simulink model "sampleModel2120_pp_532_1"  (R2021a)
settings: Solver=VariableStepAuto  StartTime=0.0  StopTime=10.0  RelTol=1e-3
undefined symbols (not defined in the file or in its folder): DiscIntNeverNeededParam, magnitude, Newton, Raphson
libraries: simulink x67, pid_lib x12
(part 2 of 3)

== system sampleModel2120_pp_532_1/emi_27 ==
  emi_34 : Inport
  Action Port : ActionPort  ActionPortLabel=if(0 > u1)
  emi_31 : Trigonometry
  emi_32 : Math  SaturateOnIntegerOverflow=on
  emi_33 : Gain
  emi_35 : Outport
  wires:
  emi_34/1 -> emi_31/1
  emi_31/1 -> emi_32/1
  emi_32/1 -> emi_33/1

== system sampleModel2120_pp_532_1/emi_45 ==
  emi_52 : Inport
  Action Port : ActionPort  ActionPortLabel=if(0 > u1)
  emi_49 : Trigonometry
  emi_50 : Abs
  emi_51 : Trigonometry
  emi_53 : Outport
  wires:
  emi_52/1 -> emi_49/1
  emi_49/1 -> emi_50/1
  emi_50/1 -> emi_51/1

== system sampleModel2120_pp_532_1/emi_6 ==
  emi_13 : Inport
  Action Port : ActionPort  ActionPortLabel=if(-1.783329e+09 > u1)
  emi_10 : Abs
  emi_11 : Gain
  emi_12 : Abs
  emi_14 : Outport
  wires:
  emi_13/1 -> emi_10/1
  emi_10/1 -> emi_11/1
  emi_11/1 -> emi_12/1

== system sampleModel2120_pp_532_1/emi_66 ==
  emi_73 : Inport
  Action Port : ActionPort  ActionPortLabel=if(0 > u1)
  emi_70 : Gain
  emi_71 : Math  SaturateOnIntegerOverflow=on
  emi_72 : Trigonometry
  emi_74 : Outport
  wires:
  emi_73/1 -> emi_70/1
  emi_70/1 -> emi_71/1
  emi_71/1 -> emi_72/1

== system sampleModel2120_pp_532_1/emi_90 ==
  emi_97 : Inport
  Action Port : ActionPort  ActionPortLabel=if(0 > u1)
  emi_94 : Abs
  emi_95 : Gain
  emi_96 : Trigonometry
  emi_98 : Outport
  wires:
  emi_97/1 -> emi_94/1
  emi_94/1 -> emi_95/1
  emi_95/1 -> emi_96/1

== system sampleModel2120_pp_532_1/cfblk45/cfblk10 ==
  cfblk1 : Inport
  cfblk10 : Sum  Inputs=+  OutDataTypeStr=double
  cfblk11 : Bias  Bias=[143732452.396222]
  cfblk3 : DiscreteFir  SampleTime=1
  cfblk4 : simulink/Discrete/Transfer Fcn Real Zero  ZeroZ=0.75  ICPrevInput=0.0  DoSatur=off
      settings: SourceProductBaseCode=SL
  cfblk5 : simulink/Discrete/Transfer Fcn First Order  PoleZ=0.95  ICPrevOutput=0.0  DoSatur=off
  cfblk6 : Delay  DelayLengthSource=Input port  SampleTime=1
      settings: InputPortMap=u0,p1
  cfblk7 : Bias  Bias=[415695908.441253]
  cfblk8 : simulink/Math Operations/Slider Gain  gain=1  low=0  high=2
  cfblk9 : Rounding
  cyemi_{24..33} (10 alike) : DataTypeConversion  OutDataTypeStr=double
  cfblk2 : Outport
  wires:
  cfblk9/1 -> cfblk2/1
  cfblk11/1 -> cyemi_26/1, cyemi_30/1
  cyemi_24/1 -> cfblk10/1
  cfblk5/1 -> cyemi_24/1
  cyemi_25/1 -> cfblk11/1
  cfblk8/1 -> cyemi_25/1
  cyemi_26/1 -> cfblk3/1
  cyemi_27/1 -> cfblk4/1
  cfblk3/1 -> cyemi_27/1
  cyemi_28/1 -> cfblk5/1
  cfblk4/1 -> cyemi_28/1
  cyemi_29/1 -> cfblk6/1
  cfblk10/1 -> cyemi_29/1
  cyemi_30/1 -> cfblk6/2
  cyemi_31/1 -> cfblk7/1
  cfblk1/1 -> cyemi_31/1
  cyemi_32/1 -> cfblk8/1
  cfblk7/1 -> cyemi_32/1
  cyemi_33/1 -> cfblk9/1
  cfblk6/1 -> cyemi_33/1

== system sampleModel2120_pp_532_1/cfblk45/cfblk11 ==
  cfblk1 : Inport
  cfblk6 : Inport  Port=2
  cfblk7 : Inport  Port=3
  cfblk8 : Inport  Port=4
  cfblk9 : Inport  Port=5
  cfblk3 : Sum  Inputs=-+  OutDataTypeStr=double
  cfblk4 : Constant  Value=[-156405987.882864]  OutDataTypeStr=double  SampleTime=1
  cfblk5 : Constant  Value=[-751982074.552397]  OutDataTypeStr=double  SampleTime=1
  cyemi_39 : DataTypeConversion  OutDataTypeStr=double
  cyemi_40 : DataTypeConversion  OutDataTypeStr=double
  cfblk2 : Outport
  cfblk10 : Outport  Port=2
  wires:
  cfblk4/1 -> cfblk10/1
  cfblk5/1 -> cfblk2/1
  cyemi_39/1 -> cfblk3/1
  cfblk8/1 -> cyemi_39/1
  cyemi_40/1 -> cfblk3/2
  cfblk7/1 -> cyemi_40/1

== system sampleModel2120_pp_532_1/cfblk45/cfblk12 ==
  cfblk1 : Inport
  cfblk11 : Inport  Port=2
  cfblk10 : Constant  Value=[257671330.793710]  OutDataTypeStr=double  SampleTime=1
  cfblk12 : Delay  SampleTime=1
  cfblk3 : simulink/Discrete/Transfer Fcn First Order  PoleZ=0.95  ICPrevOutput=0.0  DoSatur=off
  cfblk4 : Delay  ShowEnablePort=on  SampleTime=1
      settings: InputPortMap=u0,e6
  cfblk5 : DiscreteFilter  SampleTime=1
  cfblk6 : Product  OutDataTypeStr=double
  cfblk7 : Sum  Inputs=--  OutDataTypeStr=double
  cfblk8 : Sum  OutDataTypeStr=double
  cfblk9 : Constant  Value=[-533370526.019482]  OutDataTypeStr=double  SampleTime=1
  cyemi_{43..53} (11 alike) : DataTypeConversion  OutDataTypeStr=double
  cfblk2 : Outport
  wires:
  cfblk5/1 -> cfblk2/1
  cfblk1/1 -> cyemi_46/1, cyemi_50/1
  cyemi_43/1 -> cfblk12/1
  cfblk4/1 -> cyemi_43/1
  cyemi_44/1 -> cfblk3/1
  cfblk10/1 -> cyemi_44/1
  cyemi_45/1 -> cfblk4/1
  cfblk8/1 -> cyemi_45/1
  cyemi_46/1 -> cfblk4/2
  cyemi_47/1 -> cfblk5/1
  cfblk9/1 -> cyemi_47/1
  cyemi_48/1 -> cfblk6/1
  cfblk7/1 -> cyemi_48/1
  cyemi_49/1 -> cfblk6/2
  cfblk12/1 -> cyemi_49/1
  cyemi_50/1 -> cfblk7/1
  cyemi_51/1 -> cfblk7/2
  cfblk11/1 -> cyemi_51/1
  cyemi_52/1 -> cfblk8/1
  cfblk3/1 -> cyemi_52/1
  cyemi_53/1 -> cfblk8/2
  cfblk6/1 -> cyemi_53/1

== system sampleModel2120_pp_532_1/cfblk45/cfblk13 ==
  cfblk1 : Inport
  cfblk11 : Inport  Port=2
  cfblk12 : Inport  Port=3
  cfblk10 : Constant  Value=[408866745.308150]  OutDataTypeStr=double  SampleTime=1
  cfblk3 : Delay  DelayLengthSource=Input port  SampleTime=1
      settings: InputPortMap=u0,p1
  cfblk4 : Sqrt  OutDataTypeStr=double  SaturateOnIntegerOverflow=on
  cfblk5 : Sqrt  Operator=rSqrt  OutDataTypeStr=double  AlgorithmType=Newton-Raphson  SaturateOnIntegerOverflow=on
  cfblk6 : PermuteDimensions
  cfblk7 : Sum  Inputs=+  OutDataTypeStr=double
  cfblk8 : Sum  OutDataTypeStr=double
  cfblk9 : Constant  Value=[-458549736.263583]  OutDataTypeStr=double  SampleTime=1
  cyemi_{57..64} (8 alike) : DataTypeConversion  OutDataTypeStr=double
  cfblk2 : Outport
  wires:
  cfblk4/1 -> cfblk2/1
  cyemi_57/1 -> cfblk3/1
  cfblk11/1 -> cyemi_57/1
  cyemi_58/1 -> cfblk3/2
  cfblk12/1 -> cyemi_58/1
  cyemi_59/1 -> cfblk4/1
  cfblk6/1 -> cyemi_59/1
  cyemi_60/1 -> cfblk5/1
  cfblk3/1 -> cyemi_60/1
  cyemi_61/1 -> cfblk6/1
  cfblk7/1 -> cyemi_61/1
  cyemi_62/1 -> cfblk7/1
  cfblk9/1 -> cyemi_62/1
  cyemi_63/1 -> cfblk8/1
  cfblk10/1 -> cyemi_63/1
  cyemi_64/1 -> cfblk8/2
  cfblk1/1 -> cyemi_64/1

== system sampleModel2120_pp_532_1/cfblk45/cfblk14 ==
  cfblk1 : Inport
  cfblk7 : Inport  Port=2
  cfblk8 : Inport  Port=3
  cfblk3 : Delay  SampleTime=1
  cfblk4 : Delay  SampleTime=1
  cfblk5 : ComplexToRealImag
  cfblk6 : Trigonometry
  cyemi_{68..71} (4 alike) : DataTypeConversion  OutDataTypeStr=double
  cfblk2 : Outport
  cfblk9 : Outport  Port=2
  wires:
  cfblk3/1 -> cfblk2/1
  cfblk8/1 -> cfblk9/1
  cyemi_68/1 -> cfblk3/1
  cfblk5/1 -> cyemi_68/1
  cyemi_69/1 -> cfblk4/1
  cfblk5/2 -> cyemi_69/1
  cyemi_70/1 -> cfblk5/1
  cfblk6/1 -> cyemi_70/1
  cyemi_71/1 -> cfblk6/1
  cfblk7/1 -> cyemi_71/1

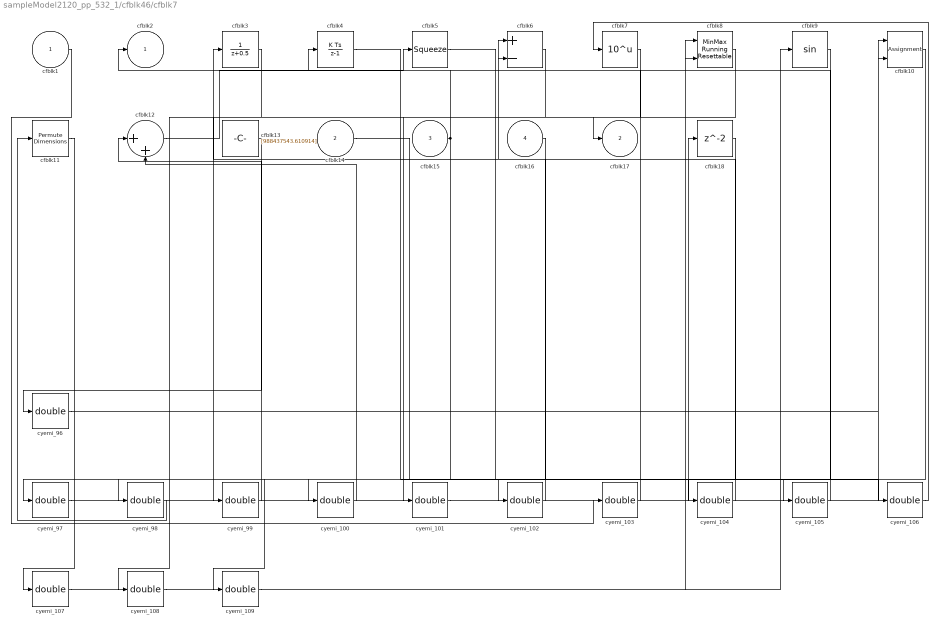
== system sampleModel2120_pp_532_1/cfblk46/cfblk7 ==
  cfblk1 : Inport
  cfblk14 : Inport  Port=2
  cfblk15 : Inport  Port=3
  cfblk16 : Inport  Port=4
  cfblk10 : Assignment  DiagnosticForDimensions=Warning  IndexOptions=Index vector (dialog)  Indices=1  OutputSizes=1
  cfblk11 : PermuteDimensions
  cfblk12 : Sum  Inputs=|++  OutDataTypeStr=double
  cfblk13 : Constant  Value=[988437543.610914]  OutDataTypeStr=double  SampleTime=1
  cfblk18 : Delay  SampleTime=1
  cfblk3 : DiscreteTransferFcn  SampleTime=1
  cfblk4 : DiscreteIntegrator  OutDataTypeStr=double  ICPrevOutput=DiscIntNeverNeededParam  ICPrevScaledInput=DiscIntNeverNeededParam
  cfblk5 : Squeeze
  cfblk6 : Sum  Inputs=+-  OutDataTypeStr=double
  cfblk7 : Math  Operator=10^u  OutDataTypeStr=double  SaturateOnIntegerOverflow=on
  cfblk8 : simulink/Math Operations/MinMax Running Resettable  Function=min  vinit=0.0
  cfblk9 : Trigonometry
  cyemi_{96..109} (14 alike) : DataTypeConversion  OutDataTypeStr=double
  cfblk2 : Outport
  cfblk17 : Outport  Port=2
  wires:
  cfblk12/1 -> cfblk5/1
  cfblk7/1 -> cfblk17/1
  cfblk15/1 -> cfblk2/1, cyemi_100/1
  cyemi_96/1 -> cfblk10/1
  cfblk13/1 -> cyemi_96/1
  cyemi_97/1 -> cfblk10/2
  cfblk16/1 -> cyemi_97/1
  cyemi_98/1 -> cfblk11/1
  cfblk3/1 -> cyemi_98/1
  cyemi_99/1 -> cfblk12/1
  cfblk8/1 -> cyemi_99/1
  cyemi_100/1 -> cfblk12/2
  cyemi_101/1 -> cfblk18/1
  cfblk6/1 -> cyemi_101/1
  cyemi_102/1 -> cfblk3/1
  cfblk9/1 -> cyemi_102/1
  cyemi_103/1 -> cfblk4/1
  cfblk1/1 -> cyemi_103/1
  cyemi_104/1 -> cfblk6/1
  cfblk14/1 -> cyemi_104/1
  cyemi_105/1 -> cfblk6/2
  cfblk5/1 -> cyemi_105/1
  cyemi_106/1 -> cfblk7/1
  cfblk4/1 -> cyemi_106/1
  cyemi_107/1 -> cfblk8/1
  cfblk11/1 -> cyemi_107/1
  cyemi_108/1 -> cfblk8/2
  cfblk18/1 -> cyemi_108/1
  cyemi_109/1 -> cfblk9/1
  cfblk10/1 -> cyemi_109/1

== system sampleModel2120_pp_532_1/cfblk47/cfblk10 ==
  cfblk1 : Inport
  cfblk13 : Inport  Port=2
  cfblk14 : Inport  Port=3
  cfblk10 : Trigonometry
  cfblk11 : Constant  Value=[893497711.855009]  OutDataTypeStr=double  SampleTime=1
  cfblk12 : Constant  Value=[-854571024.150822]  OutDataTypeStr=double  SampleTime=1
  cfblk3 : DiscreteStateSpace
  cfblk4 : Delay  DelayLengthSource=Input port  SampleTime=1
      settings: InputPortMap=u0,p1
  cfblk5 : Rounding
  cfblk6 : Sum  Inputs=|++  OutDataTypeStr=double
  cfblk7 : DotProduct  OutDataTypeStr=double  InputSameDT=on
  cfblk8 : Trigonometry
  cfblk9 : Product  Inputs=*  OutDataTypeStr=double
  cyemi_{115..125} (11 alike) : DataTypeConversion  OutDataTypeStr=double
  cfblk2 : Outport
  cfblk15 : Outport  Port=2
  wires:
  cfblk9/1 -> cfblk2/1
  cfblk10/1 -> cfblk15/1
  cyemi_115/1 -> cfblk10/1
  cfblk7/1 -> cyemi_115/1
  cyemi_116/1 -> cfblk3/1
  cfblk13/1 -> cyemi_116/1
  cyemi_117/1 -> cfblk4/1
  cfblk5/1 -> cyemi_117/1
  cyemi_118/1 -> cfblk4/2
  cfblk3/1 -> cyemi_118/1
  cyemi_119/1 -> cfblk5/1
  cfblk1/1 -> cyemi_119/1
  cyemi_120/1 -> cfblk6/1
  cfblk12/1 -> cyemi_120/1
  cyemi_121/1 -> cfblk6/2
  cfblk14/1 -> cyemi_121/1
  cyemi_122/1 -> cfblk7/1
  cfblk8/1 -> cyemi_122/1
  cyemi_123/1 -> cfblk7/2
  cfblk4/1 -> cyemi_123/1
  cyemi_124/1 -> cfblk8/1
  cfblk11/1 -> cyemi_124/1
  cyemi_125/1 -> cfblk9/1
  cfblk6/1 -> cyemi_125/1

== system sampleModel2120_pp_532_1/cfblk47/cfblk11 ==
  cfblk1 : Inport
  cfblk11 : Delay  SampleTime=1
  cfblk12 : Delay  SampleTime=1
  cfblk3 : PermuteDimensions
  cfblk4 : Product  Inputs=*  OutDataTypeStr=double
  cfblk5 : Sin  TimeSource=Use external signal  SampleTime=0
  cfblk6 : Rounding
  cfblk7 : Sum  Inputs=+  OutDataTypeStr=double
  cfblk8 : DotProduct  OutDataTypeStr=double  InputSameDT=on
  cfblk9 : Product  OutDataTypeStr=double
  cyemi_{127..137} (11 alike) : DataTypeConversion  OutDataTypeStr=double
  cfblk2 : Outport
  cfblk10 : Outport  Port=2
  wires:
  cfblk5/1 -> cyemi_133/1, cyemi_134/1
  cfblk4/1 -> cfblk10/1
  cfblk7/1 -> cyemi_128/1, cyemi_129/1
  cfblk8/1 -> cfblk2/1
  cfblk6/1 -> cyemi_127/1, cyemi_135/1
  cyemi_127/1 -> cfblk11/1
  cyemi_128/1 -> cfblk12/1
  cyemi_129/1 -> cfblk3/1
  cyemi_130/1 -> cfblk4/1
  cfblk3/1 -> cyemi_130/1
  cyemi_131/1 -> cfblk5/1
  cfblk12/1 -> cyemi_131/1
  cyemi_132/1 -> cfblk6/1
  cfblk9/1 -> cyemi_132/1
  cyemi_133/1 -> cfblk7/1
  cyemi_134/1 -> cfblk8/1
  cyemi_135/1 -> cfblk8/2
  cyemi_136/1 -> cfblk9/1
  cfblk1/1 -> cyemi_136/1
  cyemi_137/1 -> cfblk9/2
  cfblk11/1 -> cyemi_137/1

== system sampleModel2120_pp_532_1/cfblk47/cfblk12 ==
  cfblk1 : Inport
  cfblk11 : Inport  Port=2
  cfblk12 : Inport  Port=3
  cfblk13 : Inport  Port=4
  cfblk14 : Inport  Port=5
  cfblk15 : Inport  Port=6
  cfblk10 : Rounding
  cfblk16 : Delay  SampleTime=1
  cfblk3 : DiscreteFir  SampleTime=1
  cfblk4 : DiscreteFilter  SampleTime=1
  cfblk5 : simulink/Discrete/Transfer Fcn Lead or Lag  PoleZ=0.95  ZeroZ=0.75  ICPrevOutput=0.0  ICPrevInput=0.0  DoSatur=off
      settings: SourceProductBaseCode=SL
  cfblk6 : DotProduct  OutDataTypeStr=double  InputSameDT=on
  cfblk7 : Sqrt  OutDataTypeStr=double  SaturateOnIntegerOverflow=on
  cfblk8 : DotProduct  OutDataTypeStr=double  InputSameDT=on
  cfblk9 : DotProduct  OutDataTypeStr=double  InputSameDT=on
  cyemi_{144..155} (12 alike) : DataTypeConversion  OutDataTypeStr=double
  cfblk2 : Outport
  wires:
  cfblk15/1 -> cfblk2/1
  cyemi_144/1 -> cfblk10/1
  cfblk9/1 -> cyemi_144/1
  cyemi_145/1 -> cfblk16/1
  cfblk10/1 -> cyemi_145/1
  cyemi_146/1 -> cfblk3/1
  cfblk16/1 -> cyemi_146/1
  cyemi_147/1 -> cfblk4/1
  cfblk14/1 -> cyemi_147/1
  cyemi_148/1 -> cfblk5/1
  cfblk11/1 -> cyemi_148/1
  cyemi_149/1 -> cfblk6/1
  cfblk7/1 -> cyemi_149/1
  cyemi_150/1 -> cfblk6/2
  cfblk12/1 -> cyemi_150/1
  cyemi_151/1 -> cfblk7/1
  cfblk3/1 -> cyemi_151/1
  cyemi_152/1 -> cfblk8/1
  cfblk4/1 -> cyemi_152/1
  cyemi_153/1 -> cfblk8/2
  cfblk13/1 -> cyemi_153/1
  cyemi_154/1 -> cfblk9/1
  cfblk6/1 -> cyemi_154/1
  cyemi_155/1 -> cfblk9/2
  cfblk8/1 -> cyemi_155/1

== system sampleModel2120_pp_532_1/cfblk47/cfblk9 ==
  cfblk1 : Inport
  cfblk12 : Inport  Port=2
  cfblk13 : Inport  Port=3
  cfblk10 : DotProduct  OutDataTypeStr=double  InputSameDT=on
  cfblk11 : Sum  Inputs=+-  OutDataTypeStr=double
  cfblk3 : pid_lib/PID Controller  Controller=PID  Form=Parallel  TimeDomain=Discrete-time  UseExternalTs=off  SampleTime=1  IntegratorMethod=Forward Euler  FilterMethod=Forward Euler  ControllerParametersSource=internal  P=1  I=1  D=0  UseFilter=on  N=100  TunerSelectOption=Transfer Function Based (PID Tuner App)  InitialConditionSource=internal  InitialConditionForIntegrator=0  InitialConditionForFilter=0  DifferentiatorICPrevScaledInput=0  ExternalReset=none  TrackingMode=off  Kt=1  LimitOutput=off  SatLimitsSource=internal  UpperSaturationLimit=inf  LowerSaturationLimit=-inf  LinearizeAsGain=off  AntiWindupMode=none  Kb=1  POutMin=[]  POutMax=[]  IOutMin=[]  IOutMax=[]  DOutMin=[]  DOutMax=[]  NOutMin=[]  NOutMax=[]  SumOutMin=[]  SumOutMax=[]  SaturationOutMin=[]  SaturationOutMax=[]  PParamMin=[]  PParamMax=[]  IParamMin=[]  IParamMax=[]  DParamMin=[]  DParamMax=[]  NParamMin=[]  NParamMax=[]  KbParamMin=[]  KbParamMax=[]  KtParamMin=[]  KtParamMax=[]  KbOutMin=[]  KbOutMax=[]  KtOutMin=[]  KtOutMax=[]  IntegratorOutMin=[]  IntegratorOutMax=[]  FilterOutMin=[]  FilterOutMax=[]  SumI1OutMin=[]  SumI1OutMax=[]  SumI2OutMin=[]  SumI2OutMax=[]  SumI3OutMin=[]  SumI3OutMax=[]  SumI4OutMin=[]  SumI4OutMax=[]  SumDOutMin=[]  SumDOutMax=[]  DifferentiatorOutMin=[]  DifferentiatorOutMax=[]  FilterDiffOutCoefMin=[]  FilterDiffOutCoefMax=[]  ReciprocalOutMin=[]  ReciprocalOutMax=[]  SumDenOutMin=[]  SumDenOutMax=[]  SumNumOutMin=[]  SumNumOutMax=[]  DivideOutMin=[]  DivideOutMax=[]  UdiffTsProdOutMin=[]  UdiffTsProdOutMax=[]  NTsProdOutMin=[]  NTsProdOutMax=[]  UintegralTsProdOutMin=[]  UintegralTsProdOutMax=[]  UngainTsProdOutMin=[]  UngainTsProdOutMax=[]  IntegratorContinuousStateAttributes=''  IntegratorStateMustResolveToSignalObject=off  IntegratorRTWStateStorageClass=Auto  FilterContinuousStateAttributes=''  FilterStateMustResolveToSignalObject=off  FilterRTWStateStorageClass=Auto  ParallelPVariant=InternalParameters  IdealPVariant=Disabled  IVariant=InternalParameters  DVariant=InternalParameters  IntegratorVariant=Discrete  SatVariant=Disabled  AWVariant=Passthrough  PCopyVariant=Disabled  TRVariant=Disabled  FdbkBlocksVariant=Forward  IdealPFdbkVariant=Disabled  SatFdbkVariant=Disabled  DerivativeFilterVariant=ForwardEulerFilter  NVariant=InternalParameters  NCopyVariant=Disabled  FilterICVariant=InternalICsFilter  IntegratorICVariant=InternalICs  ExternalResetVariant=Disabled  TRSumVariant=Passthrough  SumFdbkVariant=Disabled  SumVariant=Sum_PID  TsampFilterVariant=InternalTs  TsampNgainVariant=Passthrough  TsampIntegralVariant=Passthrough  ExternalSaturationOutDataTypeStr=Inherit: Same as second input
  cfblk4 : simulink/Discrete/Transfer Fcn Real Zero  ZeroZ=0.75  ICPrevInput=0.0  DoSatur=off
      settings: SourceProductBaseCode=SL
  cfblk5 : simulink/Discrete/Transfer Fcn Lead or Lag  PoleZ=0.95  ZeroZ=0.75  ICPrevOutput=0.0  ICPrevInput=0.0  DoSatur=off
      settings: SourceProductBaseCode=SL
  cfblk6 : simulink/Discrete/Transfer Fcn First Order  PoleZ=0.95  ICPrevOutput=0.0  DoSatur=off
  cfblk7 : ComplexToMagnitudeAngle
  cfblk8 : Rounding
  cfblk9 : Bias  Bias=[-695140496.108146]
  cyemi_{174..184} (11 alike) : DataTypeConversion  OutDataTypeStr=double
  cfblk2 : Outport
  cfblk14 : Outport  Port=2
  wires:
  cfblk8/1 -> cfblk2/1
  cfblk10/1 -> cfblk14/1
  cyemi_174/1 -> cfblk10/1
  cfblk5/1 -> cyemi_174/1
  cyemi_175/1 -> cfblk10/2
  cfblk1/1 -> cyemi_175/1
  cyemi_176/1 -> cfblk11/1
  cfblk7/1 -> cyemi_176/1
  cyemi_177/1 -> cfblk11/2
  cfblk4/1 -> cyemi_177/1
  cyemi_178/1 -> cfblk3/1
  cfblk13/1 -> cyemi_178/1
  cyemi_179/1 -> cfblk4/1
  cfblk7/2 -> cyemi_179/1
  cyemi_180/1 -> cfblk5/1
  cfblk11/1 -> cyemi_180/1
  cyemi_181/1 -> cfblk6/1
  cfblk3/1 -> cyemi_181/1
  cyemi_182/1 -> cfblk7/1
  cfblk12/1 -> cyemi_182/1
  cyemi_183/1 -> cfblk8/1
  cfblk9/1 -> cyemi_183/1
  cyemi_184/1 -> cfblk9/1
  cfblk6/1 -> cyemi_184/1

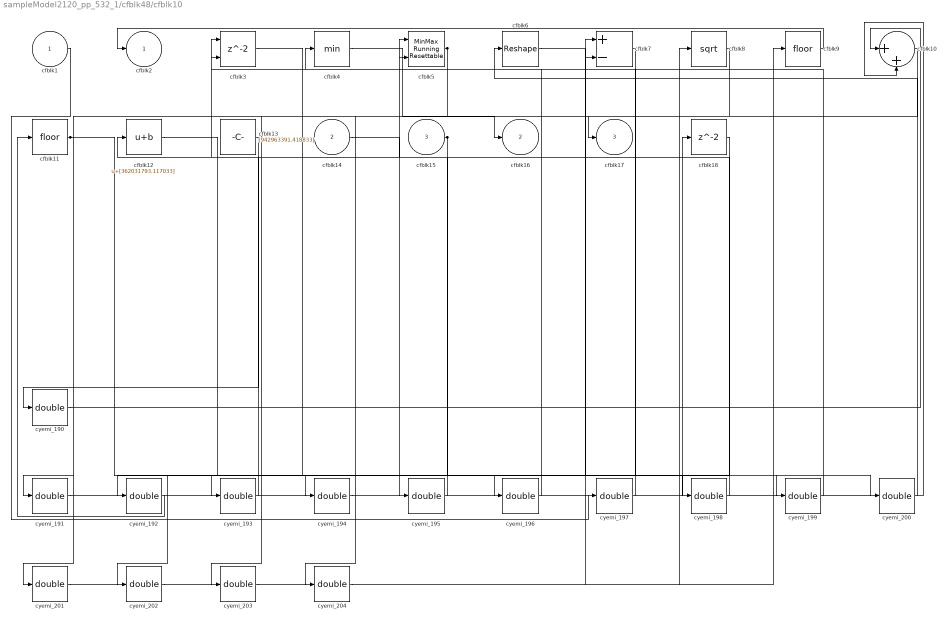
== system sampleModel2120_pp_532_1/cfblk48/cfblk10 ==
  cfblk1 : Inport
  cfblk14 : Inport  Port=2
  cfblk15 : Inport  Port=3
  cfblk10 : Sum  Inputs=|++  OutDataTypeStr=double
  cfblk11 : Rounding
  cfblk12 : Bias  Bias=[362031793.117033]
  cfblk13 : Constant  Value=[942963391.418833]  OutDataTypeStr=double  SampleTime=1
  cfblk18 : Delay  SampleTime=1
  cfblk3 : Delay  ShowEnablePort=on  SampleTime=1
      settings: InputPortMap=u0,e6
  cfblk4 : MinMax  OutDataTypeStr=double
  cfblk5 : simulink/Math Operations/MinMax Running Resettable  Function=min  vinit=0.0
  cfblk6 : Reshape
  cfblk7 : Sum  Inputs=+-  OutDataTypeStr=double
  cfblk8 : Sqrt  OutDataTypeStr=double  SaturateOnIntegerOverflow=on
  cfblk9 : Rounding
  cyemi_{190..204} (15 alike) : DataTypeConversion  OutDataTypeStr=double
  cfblk2 : Outport
  cfblk16 : Outport  Port=2
  cfblk17 : Outport  Port=3
  wires:
  cfblk10/1 -> cfblk17/1
  cfblk15/1 -> cyemi_193/1, cyemi_202/1
  cfblk11/1 -> cyemi_191/1, cyemi_194/1
  cfblk4/1 -> cfblk16/1
  cfblk5/1 -> cyemi_201/1, cyemi_203/1
  cfblk9/1 -> cfblk2/1
  cyemi_190/1 -> cfblk10/1
  cfblk13/1 -> cyemi_190/1
  cyemi_191/1 -> cfblk10/2
  cyemi_192/1 -> cfblk11/1
  cfblk7/1 -> cyemi_192/1
  cyemi_193/1 -> cfblk12/1
  cyemi_194/1 -> cfblk18/1
  cyemi_195/1 -> cfblk3/1
  cfblk14/1 -> cyemi_195/1
  cyemi_196/1 -> cfblk3/2
  cfblk18/1 -> cyemi_196/1
  cyemi_197/1 -> cfblk4/1
  cfblk1/1 -> cyemi_197/1
  cyemi_198/1 -> cfblk5/1
  cfblk6/1 -> cyemi_198/1
  cyemi_199/1 -> cfblk5/2
  cfblk12/1 -> cyemi_199/1
  cyemi_200/1 -> cfblk6/1
  cfblk3/1 -> cyemi_200/1
  cyemi_201/1 -> cfblk7/1
  cyemi_202/1 -> cfblk7/2
  cyemi_203/1 -> cfblk8/1
  cyemi_204/1 -> cfblk9/1
  cfblk8/1 -> cyemi_204/1

== system sampleModel2120_pp_532_1/cfblk48/cfblk11 ==
  cfblk1 : Inport
  cfblk7 : Inport  Port=2
  cfblk8 : Inport  Port=3
  cfblk9 : Inport  Port=4
  cfblk10 : Inport  Port=5
  cfblk3 : pid_lib/PID Controller  Controller=PID  Form=Parallel  TimeDomain=Discrete-time  UseExternalTs=off  SampleTime=1  IntegratorMethod=Forward Euler  FilterMethod=Forward Euler  ControllerParametersSource=internal  P=1  I=1  D=0  UseFilter=on  N=100  TunerSelectOption=Transfer Function Based (PID Tuner App)  InitialConditionSource=internal  InitialConditionForIntegrator=0  InitialConditionForFilter=0  DifferentiatorICPrevScaledInput=0  ExternalReset=none  TrackingMode=off  Kt=1  LimitOutput=off  SatLimitsSource=internal  UpperSaturationLimit=inf  LowerSaturationLimit=-inf  LinearizeAsGain=off  AntiWindupMode=none  Kb=1  POutMin=[]  POutMax=[]  IOutMin=[]  IOutMax=[]  DOutMin=[]  DOutMax=[]  NOutMin=[]  NOutMax=[]  SumOutMin=[]  SumOutMax=[]  SaturationOutMin=[]  SaturationOutMax=[]  PParamMin=[]  PParamMax=[]  IParamMin=[]  IParamMax=[]  DParamMin=[]  DParamMax=[]  NParamMin=[]  NParamMax=[]  KbParamMin=[]  KbParamMax=[]  KtParamMin=[]  KtParamMax=[]  KbOutMin=[]  KbOutMax=[]  KtOutMin=[]  KtOutMax=[]  IntegratorOutMin=[]  IntegratorOutMax=[]  FilterOutMin=[]  FilterOutMax=[]  SumI1OutMin=[]  SumI1OutMax=[]  SumI2OutMin=[]  SumI2OutMax=[]  SumI3OutMin=[]  SumI3OutMax=[]  SumI4OutMin=[]  SumI4OutMax=[]  SumDOutMin=[]  SumDOutMax=[]  DifferentiatorOutMin=[]  DifferentiatorOutMax=[]  FilterDiffOutCoefMin=[]  FilterDiffOutCoefMax=[]  ReciprocalOutMin=[]  ReciprocalOutMax=[]  SumDenOutMin=[]  SumDenOutMax=[]  SumNumOutMin=[]  SumNumOutMax=[]  DivideOutMin=[]  DivideOutMax=[]  UdiffTsProdOutMin=[]  UdiffTsProdOutMax=[]  NTsProdOutMin=[]  NTsProdOutMax=[]  UintegralTsProdOutMin=[]  UintegralTsProdOutMax=[]  UngainTsProdOutMin=[]  UngainTsProdOutMax=[]  IntegratorContinuousStateAttributes=''  IntegratorStateMustResolveToSignalObject=off  IntegratorRTWStateStorageClass=Auto  FilterContinuousStateAttributes=''  FilterStateMustResolveToSignalObject=off  FilterRTWStateStorageClass=Auto  ParallelPVariant=InternalParameters  IdealPVariant=Disabled  IVariant=InternalParameters  DVariant=InternalParameters  IntegratorVariant=Discrete  SatVariant=Disabled  AWVariant=Passthrough  PCopyVariant=Disabled  TRVariant=Disabled  FdbkBlocksVariant=Forward  IdealPFdbkVariant=Disabled  SatFdbkVariant=Disabled  DerivativeFilterVariant=ForwardEulerFilter  NVariant=InternalParameters  NCopyVariant=Disabled  FilterICVariant=InternalICsFilter  IntegratorICVariant=InternalICs  ExternalResetVariant=Disabled  TRSumVariant=Passthrough  SumFdbkVariant=Disabled  SumVariant=Sum_PID  TsampFilterVariant=InternalTs  TsampNgainVariant=Passthrough  TsampIntegralVariant=Passthrough  ExternalSaturationOutDataTypeStr=Inherit: Same as second input
  cfblk4 : simulink/Discrete/Transfer Fcn Real Zero  ZeroZ=0.75  ICPrevInput=0.0  DoSatur=off
      settings: SourceProductBaseCode=SL
  cfblk5 : simulink/Discrete/Transfer Fcn First Order  PoleZ=0.95  ICPrevOutput=0.0  DoSatur=off
  cfblk6 : simulink/Discrete/Transfer Fcn Lead or Lag  PoleZ=0.95  ZeroZ=0.75  ICPrevOutput=0.0  ICPrevInput=0.0  DoSatur=off
      settings: SourceProductBaseCode=SL
  cyemi_{210..213} (4 alike) : DataTypeConversion  OutDataTypeStr=double
  cfblk2 : Outport
  cfblk11 : Outport  Port=2
  wires:
  cfblk1/1 -> cfblk11/1
  cfblk6/1 -> cfblk2/1
  cyemi_210/1 -> cfblk3/1
  cfblk10/1 -> cyemi_210/1
  cyemi_211/1 -> cfblk4/1
  cfblk7/1 -> cyemi_211/1
  cyemi_212/1 -> cfblk5/1
  cfblk9/1 -> cyemi_212/1
  cyemi_213/1 -> cfblk6/1
  cfblk5/1 -> cyemi_213/1

== system sampleModel2120_pp_532_1/cfblk48/cfblk12 ==
  cfblk1 : Inport
  cfblk8 : Inport  Port=2
  cfblk9 : Inport  Port=3
  cfblk3 : Sin  TimeSource=Use external signal  SampleTime=0
  cfblk4 : Trigonometry
  cfblk5 : Abs  OutDataTypeStr=double
  cfblk6 : Constant  Value=[518719100.670352]  OutDataTypeStr=double  SampleTime=1
  cfblk7 : Constant  Value=[188716034.408801]  OutDataTypeStr=double  SampleTime=1
  cyemi_217 : DataTypeConversion  OutDataTypeStr=double
  cyemi_218 : DataTypeConversion  OutDataTypeStr=double
  cyemi_219 : DataTypeConversion  OutDataTypeStr=double
  cfblk2 : Outport
  cfblk10 : Outport  Port=2
  wires:
  cfblk8/1 -> cfblk10/1
  cfblk9/1 -> cfblk2/1
  cyemi_217/1 -> cfblk3/1
  cfblk5/1 -> cyemi_217/1
  cyemi_218/1 -> cfblk4/1
  cfblk6/1 -> cyemi_218/1
  cyemi_219/1 -> cfblk5/1
  cfblk4/1 -> cyemi_219/1

== system sampleModel2120_pp_532_1/cfblk49/cfblk49 ==
  cfblk1 : Inport
  cfblk{8..12} (5 alike) : Delay  SampleTime=1
  cfblk3 : Polyval  Coefs=[ +2.081618890e-019, -1.441693666e-014, +4.719686976e-010, -8.536869453e-006, +1.621573104e-001, -8.087801117e+001 ]
  cfblk4 : Reshape
  cfblk5 : Subsystem
  cfblk6 : Subsystem
  cfblk7 : Subsystem
  cyemi_{229..235,241..245,253..255,264..265} (17 alike) : DataTypeConversion  OutDataTypeStr=double
  cfblk2 : Outport
  wires:
  cyemi_265/1 -> cfblk9/1
  cyemi_264/1 -> cfblk8/1
  cfblk12/1 -> cyemi_255/1
  cyemi_255/1 -> cfblk7/3(cfblk13)
  cfblk6/4(cfblk17) -> cyemi_254/1
  cyemi_254/1 -> cfblk7/2(cfblk12)
  cfblk6/2(cfblk15) -> cyemi_253/1
  cyemi_253/1 -> cfblk7/1(cfblk1)
  cfblk9/1 -> cyemi_245/1
  cyemi_245/1 -> cfblk6/5(cfblk14)
  cfblk11/1 -> cyemi_244/1
  cyemi_244/1 -> cfblk6/4(cfblk13)
  cfblk10/1 -> cyemi_243/1
  cyemi_243/1 -> cfblk6/3(cfblk12)
  cfblk1/1 -> cyemi_242/1
  cyemi_242/1 -> cfblk6/2(cfblk11)
  cfblk8/1 -> cyemi_241/1
  cyemi_241/1 -> cfblk6/1(cfblk1)
  cfblk6/3(cfblk16) -> cyemi_235/1
  cyemi_235/1 -> cfblk5/2(cfblk7)
  cfblk7/1(cfblk2) -> cyemi_234/1
  cyemi_234/1 -> cfblk5/1(cfblk1)
  cyemi_233/1 -> cfblk4/1
  cfblk6/1(cfblk2) -> cyemi_232/1
  cyemi_232/1 -> cfblk3/1
  cyemi_231/1 -> cfblk12/1
  cyemi_230/1 -> cfblk11/1
  cyemi_229/1 -> cfblk10/1
  cfblk5/1(cfblk2) -> cyemi_231/1, cyemi_230/1, cfblk2/1
  cfblk4/1 -> cyemi_265/1, cyemi_264/1
  cfblk3/1 -> cyemi_233/1, cyemi_229/1

== system sampleModel2120_pp_532_1/cfblk51/cfblk10 ==
  cfblk1 : Inport
  cfblk11 : Inport  Port=2
  cfblk12 : Inport  Port=3
  cfblk13 : Inport  Port=4
  cfblk14 : Inport  Port=5
  cfblk15 : Inport  Port=6
  cfblk10 : Constant  Value=[-260520393.744938]  OutDataTypeStr=double  SampleTime=1
  cfblk3 : Delay  DelayLengthSource=Input port  SampleTime=1
      settings: InputPortMap=u0,p1
  cfblk4 : Rounding
  cfblk5 : Abs  OutDataTypeStr=double
  cfblk6 : Sqrt  OutDataTypeStr=double  SaturateOnIntegerOverflow=on
  cfblk7 : Sum  Inputs=|++  OutDataTypeStr=double
  cfblk8 : Sum  Inputs=|++  OutDataTypeStr=double
  cfblk9 : Sqrt  Operator=rSqrt  OutDataTypeStr=double  AlgorithmType=Newton-Raphson  SaturateOnIntegerOverflow=on
  cyemi_{281..290} (10 alike) : DataTypeConversion  OutDataTypeStr=double
  cfblk2 : Outport
  cfblk16 : Outport  Port=2
  cfblk17 : Outport  Port=3
  wires:
  cfblk13/1 -> cfblk17/1
  cfblk15/1 -> cfblk16/1
  cfblk9/1 -> cfblk2/1
  cyemi_281/1 -> cfblk3/1
  cfblk12/1 -> cyemi_281/1
  cyemi_282/1 -> cfblk3/2
  cfblk4/1 -> cyemi_282/1
  cyemi_283/1 -> cfblk4/1
  cfblk5/1 -> cyemi_283/1
  cyemi_284/1 -> cfblk5/1
  cfblk7/1 -> cyemi_284/1
  cyemi_285/1 -> cfblk6/1
  cfblk8/1 -> cyemi_285/1
  cyemi_286/1 -> cfblk7/1
  cfblk1/1 -> cyemi_286/1
  cyemi_287/1 -> cfblk7/2
  cfblk6/1 -> cyemi_287/1
  cyemi_288/1 -> cfblk8/1
  cfblk11/1 -> cyemi_288/1
  cyemi_289/1 -> cfblk8/2
  cfblk14/1 -> cyemi_289/1
  cyemi_290/1 -> cfblk9/1
  cfblk10/1 -> cyemi_290/1

== system sampleModel2120_pp_532_1/cfblk51/cfblk9 ==
  cfblk1 : Inport
  cfblk9 : Inport  Port=2
  cfblk10 : Inport  Port=3
  cfblk11 : Inport  Port=4
  cfblk12 : Inport  Port=5
  cfblk13 : Inport  Port=6
  cfblk15 : Delay  SampleTime=1
  cfblk3 : pid_lib/PID Controller  Controller=PID  Form=Parallel  TimeDomain=Discrete-time  UseExternalTs=off  SampleTime=1  IntegratorMethod=Forward Euler  FilterMethod=Forward Euler  ControllerParametersSource=internal  P=1  I=1  D=0  UseFilter=on  N=100  TunerSelectOption=Transfer Function Based (PID Tuner App)  InitialConditionSource=internal  InitialConditionForIntegrator=0  InitialConditionForFilter=0  DifferentiatorICPrevScaledInput=0  ExternalReset=none  TrackingMode=off  Kt=1  LimitOutput=off  SatLimitsSource=internal  UpperSaturationLimit=inf  LowerSaturationLimit=-inf  LinearizeAsGain=off  AntiWindupMode=none  Kb=1  POutMin=[]  POutMax=[]  IOutMin=[]  IOutMax=[]  DOutMin=[]  DOutMax=[]  NOutMin=[]  NOutMax=[]  SumOutMin=[]  SumOutMax=[]  SaturationOutMin=[]  SaturationOutMax=[]  PParamMin=[]  PParamMax=[]  IParamMin=[]  IParamMax=[]  DParamMin=[]  DParamMax=[]  NParamMin=[]  NParamMax=[]  KbParamMin=[]  KbParamMax=[]  KtParamMin=[]  KtParamMax=[]  KbOutMin=[]  KbOutMax=[]  KtOutMin=[]  KtOutMax=[]  IntegratorOutMin=[]  IntegratorOutMax=[]  FilterOutMin=[]  FilterOutMax=[]  SumI1OutMin=[]  SumI1OutMax=[]  SumI2OutMin=[]  SumI2OutMax=[]  SumI3OutMin=[]  SumI3OutMax=[]  SumI4OutMin=[]  SumI4OutMax=[]  SumDOutMin=[]  SumDOutMax=[]  DifferentiatorOutMin=[]  DifferentiatorOutMax=[]  FilterDiffOutCoefMin=[]  FilterDiffOutCoefMax=[]  ReciprocalOutMin=[]  ReciprocalOutMax=[]  SumDenOutMin=[]  SumDenOutMax=[]  SumNumOutMin=[]  SumNumOutMax=[]  DivideOutMin=[]  DivideOutMax=[]  UdiffTsProdOutMin=[]  UdiffTsProdOutMax=[]  NTsProdOutMin=[]  NTsProdOutMax=[]  UintegralTsProdOutMin=[]  UintegralTsProdOutMax=[]  UngainTsProdOutMin=[]  UngainTsProdOutMax=[]  IntegratorContinuousStateAttributes=''  IntegratorStateMustResolveToSignalObject=off  IntegratorRTWStateStorageClass=Auto  FilterContinuousStateAttributes=''  FilterStateMustResolveToSignalObject=off  FilterRTWStateStorageClass=Auto  ParallelPVariant=InternalParameters  IdealPVariant=Disabled  IVariant=InternalParameters  DVariant=InternalParameters  IntegratorVariant=Discrete  SatVariant=Disabled  AWVariant=Passthrough  PCopyVariant=Disabled  TRVariant=Disabled  FdbkBlocksVariant=Forward  IdealPFdbkVariant=Disabled  SatFdbkVariant=Disabled  DerivativeFilterVariant=ForwardEulerFilter  NVariant=InternalParameters  NCopyVariant=Disabled  FilterICVariant=InternalICsFilter  IntegratorICVariant=InternalICs  ExternalResetVariant=Disabled  TRSumVariant=Passthrough  SumFdbkVariant=Disabled  SumVariant=Sum_PID  TsampFilterVariant=InternalTs  TsampNgainVariant=Passthrough  TsampIntegralVariant=Passthrough  ExternalSaturationOutDataTypeStr=Inherit: Same as second input
  cfblk4 : DiscreteFilter  SampleTime=1
  cfblk5 : Sum  Inputs=+  OutDataTypeStr=double
  cfblk6 : Sqrt  OutDataTypeStr=double  SaturateOnIntegerOverflow=on
  cfblk7 : simulink/Math Operations/MinMax Running Resettable  Function=min  vinit=0.0
  cfblk8 : Product  Inputs=*  OutDataTypeStr=double
  cyemi_{308..315} (8 alike) : DataTypeConversion  OutDataTypeStr=double
  cfblk2 : Outport
  cfblk14 : Outport  Port=2
  wires:
  cfblk7/1 -> cfblk2/1
  cfblk9/1 -> cfblk14/1
  cyemi_308/1 -> cfblk15/1
  cfblk4/1 -> cyemi_308/1
  cyemi_309/1 -> cfblk3/1
  cfblk15/1 -> cyemi_309/1
  cyemi_310/1 -> cfblk4/1
  cfblk6/1 -> cyemi_310/1
  cyemi_311/1 -> cfblk5/1
  cfblk1/1 -> cyemi_311/1
  cyemi_312/1 -> cfblk6/1
  cfblk3/1 -> cyemi_312/1
  cyemi_313/1 -> cfblk7/1
  cfblk10/1 -> cyemi_313/1
  cyemi_314/1 -> cfblk7/2
  cfblk12/1 -> cyemi_314/1
  cyemi_315/1 -> cfblk8/1
  cfblk13/1 -> cyemi_315/1

== system sampleModel2120_pp_532_1/cfblk52/cfblk14 ==
  cfblk1 : Inport
  cfblk14 : Inport  Port=2
  cfblk15 : Inport  Port=3
  cfblk16 : Inport  Port=4
  cfblk17 : Inport  Port=5
  cfblk10 : Signum
  cfblk11 : Polyval  Coefs=[ +2.081618890e-019, -1.441693666e-014, +4.719686976e-010, -8.536869453e-006, +1.621573104e-001, -8.087801117e+001 ]
  cfblk12 : Constant  Value=[337621916.276364]  OutDataTypeStr=double  SampleTime=1
  cfblk13 : Constant  Value=[-862050304.070711]  OutDataTypeStr=double  SampleTime=1
  cfblk18 : Delay  SampleTime=1
  cfblk3 : Delay  DelayLengthSource=Input port  SampleTime=1
      settings: InputPortMap=u0,p1
  cfblk4 : Sqrt  OutDataTypeStr=double  SaturateOnIntegerOverflow=on
  cfblk5 : Product  Inputs=**  OutDataTypeStr=double
  cfblk6 : Reshape
  cfblk7 : simulink/Math Operations/Slider Gain  gain=1  low=0  high=2
  cfblk8 : UnaryMinus
  cfblk9 : Math  Operator=transpose  OutDataTypeStr=double  SaturateOnIntegerOverflow=on
  cyemi_{327..338} (12 alike) : DataTypeConversion  OutDataTypeStr=double
  cfblk2 : Outport
  wires:
  cfblk14/1 -> cfblk2/1
  cyemi_327/1 -> cfblk10/1
  cfblk17/1 -> cyemi_327/1
  cyemi_328/1 -> cfblk11/1
  cfblk6/1 -> cyemi_328/1
  cyemi_329/1 -> cfblk18/1
  cfblk8/1 -> cyemi_329/1
  cyemi_330/1 -> cfblk3/1
  cfblk13/1 -> cyemi_330/1
  cyemi_331/1 -> cfblk3/2
  cfblk15/1 -> cyemi_331/1
  cyemi_332/1 -> cfblk4/1
  cfblk16/1 -> cyemi_332/1
  cyemi_333/1 -> cfblk5/1
  cfblk1/1 -> cyemi_333/1
  cyemi_334/1 -> cfblk5/2
  cfblk3/1 -> cyemi_334/1
  cyemi_335/1 -> cfblk6/1
  cfblk18/1 -> cyemi_335/1
  cyemi_336/1 -> cfblk7/1
  cfblk12/1 -> cyemi_336/1
  cyemi_337/1 -> cfblk8/1
  cfblk11/1 -> cyemi_337/1
  cyemi_338/1 -> cfblk9/1
  cfblk5/1 -> cyemi_338/1

== system sampleModel2120_pp_532_1/cfblk53/cfblk3 ==
  cfblk1 : Inport
  cfblk9 : Inport  Port=2
  cfblk3 : simulink/Discrete/Tapped Delay  vinit=0.0  samptime=-1  NumDelays=1  DelayOrder=Oldest  includeCurrent=off
  cfblk4 : DiscreteZeroPole  Poles=[0 0.5]  Gain=1
  cfblk5 : Delay  DelayLengthSource=Input port  SampleTime=1
      settings: InputPortMap=u0,p1
  cfblk6 : simulink/Math Operations/Slider Gain  gain=1  low=0  high=2
  cfblk7 : simulink/Math Operations/MinMax Running Resettable  Function=min  vinit=0.0
  cfblk8 : simulink/Math Operations/MinMax Running Resettable  Function=min  vinit=0.0
  cyemi_{351..359} (9 alike) : DataTypeConversion  OutDataTypeStr=double
  cfblk2 : Outport
  cfblk10 : Outport  Port=2
  cfblk11 : Outport  Port=3
  cfblk12 : Outport  Port=4
  cfblk13 : Outport  Port=5
  wires:
  cfblk9/1 -> cyemi_354/1, cyemi_355/1
  cfblk6/1 -> cfblk13/1, cyemi_353/1
  cfblk3/1 -> cfblk10/1, cyemi_352/1, cyemi_359/1
  cfblk1/1 -> cfblk2/1, cfblk12/1, cyemi_358/1
  cfblk7/1 -> cfblk11/1
  cyemi_351/1 -> cfblk3/1
  cfblk5/1 -> cyemi_351/1
  cyemi_352/1 -> cfblk4/1
  cyemi_353/1 -> cfblk5/1
  cyemi_354/1 -> cfblk5/2
  cyemi_355/1 -> cfblk6/1
  cyemi_356/1 -> cfblk7/1
  cfblk8/1 -> cyemi_356/1
  cyemi_357/1 -> cfblk7/2
  cfblk4/1 -> cyemi_357/1
  cyemi_358/1 -> cfblk8/1
  cyemi_359/1 -> cfblk8/2

== system sampleModel2120_pp_532_1/cfblk53/cfblk4 ==
  cfblk1 : Inport
  cfblk8 : Inport  Port=2
  cfblk9 : Inport  Port=3
  cfblk10 : Delay  SampleTime=1
  cfblk3 : simulink/Discrete/Tapped Delay  vinit=0.0  samptime=-1  NumDelays=1  DelayOrder=Oldest  includeCurrent=off
  cfblk4 : Delay  ShowEnablePort=on  SampleTime=1
      settings: InputPortMap=u0,e6
  cfblk5 : Sqrt  Operator=rSqrt  OutDataTypeStr=double  AlgorithmType=Newton-Raphson  SaturateOnIntegerOverflow=on
  cfblk6 : Rounding
  cfblk7 : UnaryMinus
  cyemi_{363..369} (7 alike) : DataTypeConversion  OutDataTypeStr=double
  cfblk2 : Outport
  wires:
  cfblk4/1 -> cfblk2/1
  cyemi_363/1 -> cfblk10/1
  cfblk6/1 -> cyemi_363/1
  cyemi_364/1 -> cfblk3/1
  cfblk10/1 -> cyemi_364/1
  cyemi_365/1 -> cfblk4/1
  cfblk9/1 -> cyemi_365/1
  cyemi_366/1 -> cfblk4/2
  cfblk1/1 -> cyemi_366/1
  cyemi_367/1 -> cfblk5/1
  cfblk3/1 -> cyemi_367/1
  cyemi_368/1 -> cfblk6/1
  cfblk7/1 -> cyemi_368/1
  cyemi_369/1 -> cfblk7/1
  cfblk5/1 -> cyemi_369/1

== system sampleModel2120_pp_532_1/cfblk54/cfblk6 ==
  cfblk1 : Inport
  cfblk9 : Inport  Port=2
  cfblk10 : Inport  Port=3
  cfblk11 : Inport  Port=4
  cfblk12 : Inport  Port=5
  cfblk3 : UnitDelay  HasFrameUpgradeWarning=on
  cfblk4 : DiscreteTransferFcn  SampleTime=1
  cfblk5 : Polyval  Coefs=[ +2.081618890e-019, -1.441693666e-014, +4.719686976e-010, -8.536869453e-006, +1.621573104e-001, -8.087801117e+001 ]
  cfblk6 : Bias  Bias=[957126973.836130]
  cfblk7 : Sin  TimeSource=Use external signal  SampleTime=0
  cfblk8 : Constant  Value=[452018806.850211]  OutDataTypeStr=double  SampleTime=1
  cyemi_{382..386} (5 alike) : DataTypeConversion  OutDataTypeStr=double
  cfblk2 : Outport
  wires:
  cfblk4/1 -> cfblk2/1
  cyemi_382/1 -> cfblk3/1
  cfblk11/1 -> cyemi_382/1
  cyemi_383/1 -> cfblk4/1
  cfblk6/1 -> cyemi_383/1
  cyemi_384/1 -> cfblk5/1
  cfblk3/1 -> cyemi_384/1
  cyemi_385/1 -> cfblk6/1
  cfblk9/1 -> cyemi_385/1
  cyemi_386/1 -> cfblk7/1
  cfblk8/1 -> cyemi_386/1

== system sampleModel2120_pp_532_1/cfblk54/cfblk7 ==
  cfblk1 : Inport
  cfblk10 : Sqrt  OutDataTypeStr=double  SaturateOnIntegerOverflow=on
  cfblk3 : DiscreteStateSpace
  cfblk4 : Squeeze
  cfblk5 : Abs  OutDataTypeStr=double
  cfblk6 : Sqrt  OutDataTypeStr=double  SaturateOnIntegerOverflow=on
  cfblk7 : MinMax  Inputs=2  OutDataTypeStr=double
  cfblk8 : Gain  Gain=[34775156.777918]  OutDataTypeStr=double
  cfblk9 : ComplexToRealImag
  cyemi_{388..395} (8 alike) : DataTypeConversion  OutDataTypeStr=double
  cfblk2 : Outport
  wires:
  cfblk4/1 -> cfblk2/1
  cfblk1/1 -> cyemi_393/1, cyemi_395/1
  cfblk10/1 -> cfblk4/1
  cyemi_388/1 -> cfblk10/1
  cfblk5/1 -> cyemi_388/1
  cyemi_389/1 -> cfblk3/1
  cfblk9/1 -> cyemi_389/1
  cyemi_390/1 -> cfblk5/1
  cfblk8/1 -> cyemi_390/1
  cyemi_391/1 -> cfblk6/1
  cfblk9/2 -> cyemi_391/1
  cyemi_392/1 -> cfblk7/1
  cfblk3/1 -> cyemi_392/1
  cyemi_393/1 -> cfblk7/2
  cyemi_394/1 -> cfblk8/1
  cfblk6/1 -> cyemi_394/1
  cyemi_395/1 -> cfblk9/1

== system sampleModel2120_pp_532_1/cfblk54/cfblk8 ==
  cfblk1 : Inport
  cfblk10 : Delay  SampleTime=1
  cfblk11 : Delay  SampleTime=1
  cfblk3 : DiscreteIntegrator  OutDataTypeStr=double  ICPrevOutput=DiscIntNeverNeededParam  ICPrevScaledInput=DiscIntNeverNeededParam
  cfblk4 : DiscreteTransferFcn  SampleTime=1
  cfblk5 : UnitDelay  HasFrameUpgradeWarning=on
  cfblk6 : Signum
  cfblk7 : ComplexToMagnitudeAngle
  cfblk8 : MinMax  Function=max  Inputs=2  OutDataTypeStr=double
  cfblk9 : DotProduct  OutDataTypeStr=double  InputSameDT=on
  cyemi_{397..407} (11 alike) : DataTypeConversion  OutDataTypeStr=double
  cfblk2 : Outport
  wires:
  cfblk4/1 -> cfblk2/1, cyemi_398/1
  cyemi_397/1 -> cfblk10/1
  cfblk7/1 -> cyemi_397/1
  cyemi_398/1 -> cfblk11/1
  cyemi_399/1 -> cfblk3/1
  cfblk1/1 -> cyemi_399/1
  cyemi_400/1 -> cfblk4/1
  cfblk6/1 -> cyemi_400/1
  cyemi_401/1 -> cfblk5/1
  cfblk9/1 -> cyemi_401/1
  cyemi_402/1 -> cfblk6/1
  cfblk8/1 -> cyemi_402/1
  cyemi_403/1 -> cfblk7/1
  cfblk5/1 -> cyemi_403/1
  cyemi_404/1 -> cfblk8/1
  cfblk7/2 -> cyemi_404/1
  cyemi_405/1 -> cfblk8/2
  cfblk11/1 -> cyemi_405/1
  cyemi_406/1 -> cfblk9/1
  cfblk3/1 -> cyemi_406/1
  cyemi_407/1 -> cfblk9/2
  cfblk10/1 -> cyemi_407/1

== system sampleModel2120_pp_532_1/cfblk54/cfblk9 ==
  cfblk1 : Inport
  cfblk7 : Inport  Port=2
  cfblk3 : Squeeze
  cfblk4 : Squeeze
  cfblk5 : PermuteDimensions
  cfblk6 : simulink/Math Operations/MinMax Running Resettable  Function=min  vinit=0.0
  cyemi_410 : DataTypeConversion  OutDataTypeStr=double
  cyemi_411 : DataTypeConversion  OutDataTypeStr=double
  cyemi_412 : DataTypeConversion  OutDataTypeStr=double
  cfblk2 : Outport
  cfblk8 : Outport  Port=2
  cfblk9 : Outport  Port=3
  wires:
  cfblk3/1 -> cfblk4/1, cyemi_410/1
  cfblk1/1 -> cfblk3/1
  cfblk6/1 -> cfblk8/1
  cfblk5/1 -> cfblk2/1, cfblk9/1
  cyemi_410/1 -> cfblk5/1
  cyemi_411/1 -> cfblk6/1
  cfblk4/1 -> cyemi_411/1
  cyemi_412/1 -> cfblk6/2
  cfblk7/1 -> cyemi_412/1

== system sampleModel2120_pp_532_1/cfblk55/cfblk7 ==
  cfblk1 : Inport
  cfblk7 : Inport  Port=2
  cfblk8 : Inport  Port=3
  cfblk9 : Inport  Port=4
  cfblk3 : pid_lib/PID Controller (2DOF)  Controller=PID  Form=Parallel  TimeDomain=Discrete-time  UseExternalTs=off  SampleTime=1  IntegratorMethod=Forward Euler  FilterMethod=Forward Euler  ControllerParametersSource=internal  P=1  I=1  D=0  UseFilter=on  N=100  b=1  c=1  TunerSelectOption=Transfer Function Based (PID Tuner App)  InitialConditionSource=internal  InitialConditionForIntegrator=0  InitialConditionForFilter=0  DifferentiatorICPrevScaledInput=0  ExternalReset=none  TrackingMode=off  Kt=1  LimitOutput=off  SatLimitsSource=internal  UpperSaturationLimit=inf  LowerSaturationLimit=-inf  LinearizeAsGain=off  AntiWindupMode=none  Kb=1  POutMin=[]  POutMax=[]  IOutMin=[]  IOutMax=[]  DOutMin=[]  DOutMax=[]  NOutMin=[]  NOutMax=[]  bOutMin=[]  bOutMax=[]  cOutMin=[]  cOutMax=[]  SumOutMin=[]  SumOutMax=[]  SaturationOutMin=[]  SaturationOutMax=[]  PParamMin=[]  PParamMax=[]  IParamMin=[]  IParamMax=[]  DParamMin=[]  DParamMax=[]  NParamMin=[]  NParamMax=[]  bParamMin=[]  bParamMax=[]  cParamMin=[]  cParamMax=[]  KbParamMin=[]  KbParamMax=[]  KtParamMin=[]  KtParamMax=[]  KbOutMin=[]  KbOutMax=[]  KtOutMin=[]  KtOutMax=[]  IntegratorOutMin=[]  IntegratorOutMax=[]  FilterOutMin=[]  FilterOutMax=[]  SumI1OutMin=[]  SumI1OutMax=[]  SumI2OutMin=[]  SumI2OutMax=[]  SumI3OutMin=[]  SumI3OutMax=[]  SumI4OutMin=[]  SumI4OutMax=[]  SumDOutMin=[]  SumDOutMax=[]  Sum1OutMin=[]  Sum1OutMax=[]  Sum2OutMin=[]  Sum2OutMax=[]  Sum3OutMin=[]  Sum3OutMax=[]  DifferentiatorOutMin=[]  DifferentiatorOutMax=[]  FilterDiffOutCoefMin=[]  FilterDiffOutCoefMax=[]  ReciprocalOutMin=[]  ReciprocalOutMax=[]  SumDenOutMin=[]  SumDenOutMax=[]  SumNumOutMin=[]  SumNumOutMax=[]  DivideOutMin=[]  DivideOutMax=[]  UdiffTsProdOutMin=[]  UdiffTsProdOutMax=[]  NTsProdOutMin=[]  NTsProdOutMax=[]  UintegralTsProdOutMin=[]  UintegralTsProdOutMax=[]  UngainTsProdOutMin=[]  UngainTsProdOutMax=[]  IntegratorContinuousStateAttributes=''  IntegratorStateMustResolveToSignalObject=off  IntegratorRTWStateStorageClass=Auto  FilterContinuousStateAttributes=''  FilterStateMustResolveToSignalObject=off  FilterRTWStateStorageClass=Auto  ParallelPVariant=InternalParameters  IdealPVariant=Disabled  IVariant=InternalParameters  DVariant=InternalParameters  bVariant=InternalParameters  cVariant=InternalParameters  IntegratorVariant=Discrete  SatVariant=Disabled  AWVariant=Passthrough  PCopyVariant=Disabled  TRVariant=Disabled  FdbkBlocksVariant=Forward  IdealPFdbkVariant=Disabled  SatFdbkVariant=Disabled  DerivativeFilterVariant=ForwardEulerFilter  NVariant=InternalParameters  NCopyVariant=Disabled  FilterICVariant=InternalICsFilter  IntegratorICVariant=InternalICs  ExternalResetVariant=Disabled  TRSumVariant=Passthrough  SumFdbkVariant=Disabled  SumVariant=Sum_PID  TsampFilterVariant=InternalTs  TsampNgainVariant=Passthrough  TsampIntegralVariant=Passthrough  ExternalSaturationOutDataTypeStr=Inherit: Same as second input
      settings: SourceProductBaseCode=SL
  cfblk4 : Sqrt  Operator=rSqrt  OutDataTypeStr=double  AlgorithmType=Newton-Raphson  SaturateOnIntegerOverflow=on
  cfblk5 : ComplexToRealImag
  cfblk6 : Product  OutDataTypeStr=double
  cyemi_{428..433} (6 alike) : DataTypeConversion  OutDataTypeStr=double
  cfblk2 : Outport
  wires:
  cfblk3/1 -> cfblk2/1
  cyemi_428/1 -> cfblk3/1
  cfblk4/1 -> cyemi_428/1
  cyemi_429/1 -> cfblk3/2
  cfblk7/1 -> cyemi_429/1
  cyemi_430/1 -> cfblk4/1
  cfblk8/1 -> cyemi_430/1
  cyemi_431/1 -> cfblk5/1
  cfblk1/1 -> cyemi_431/1
  cyemi_432/1 -> cfblk6/1
  cfblk5/1 -> cyemi_432/1
  cyemi_433/1 -> cfblk6/2
  cfblk9/1 -> cyemi_433/1

== system sampleModel2120_pp_532_1/cfblk55/cfblk8 ==
  cfblk1 : Inport
  cfblk10 : Inport  Port=2
  cfblk11 : Inport  Port=3
  cfblk14 : Delay  SampleTime=1
  cfblk3 : DiscreteFilter  SampleTime=1
  cfblk4 : Sum  Inputs=|++  OutDataTypeStr=double
  cfblk5 : Gain  Gain=[337280846.532053]  OutDataTypeStr=double
  cfblk6 : Product  Inputs=**  OutDataTypeStr=double
  cfblk7 : Assignment  DiagnosticForDimensions=Warning  IndexOptions=Index vector (dialog)  Indices=1  OutputSizes=1
  cfblk8 : Constant  Value=[200359115.513683]  OutDataTypeStr=double  SampleTime=1
  cfblk9 : Constant  Value=[513452946.668937]  OutDataTypeStr=double  SampleTime=1
  cyemi_{437..445} (9 alike) : DataTypeConversion  OutDataTypeStr=double
  cfblk2 : Outport
  cfblk12 : Outport  Port=2
  cfblk13 : Outport  Port=3
  wires:
  cfblk1/1 -> cfblk13/1
  cfblk4/1 -> cfblk12/1
  cfblk6/1 -> cyemi_437/1, cyemi_445/1
  cfblk10/1 -> cfblk2/1
  cyemi_437/1 -> cfblk14/1
  cyemi_438/1 -> cfblk3/1
  cfblk14/1 -> cyemi_438/1
  cyemi_439/1 -> cfblk4/1
  cfblk7/1 -> cyemi_439/1
  cyemi_440/1 -> cfblk4/2
  cfblk5/1 -> cyemi_440/1
  cyemi_441/1 -> cfblk5/1
  cfblk9/1 -> cyemi_441/1
  cyemi_442/1 -> cfblk6/1
  cfblk3/1 -> cyemi_442/1
  cyemi_443/1 -> cfblk6/2
  cfblk11/1 -> cyemi_443/1
  cyemi_444/1 -> cfblk7/1
  cfblk8/1 -> cyemi_444/1
  cyemi_445/1 -> cfblk7/2

== system sampleModel2120_pp_532_1/cfblk55/cfblk9 ==
  cfblk1 : Inport
  cfblk12 : Inport  Port=2
  cfblk13 : Inport  Port=3
  cfblk14 : Inport  Port=4
  cfblk10 : Signum
  cfblk11 : Constant  Value=[-925199390.932375]  OutDataTypeStr=double  SampleTime=1
  cfblk17 : Delay  SampleTime=1
  cfblk3 : simulink/Discrete/Difference  ICPrevInput=0.0  OutMin=[]  OutMax=[]  OutDataTypeStr=double  OutputDataTypeScalingMode=double  OutDataType=fixdt(1, 16)  OutScaling=2^-10  DoSatur=off
  cfblk4 : Delay  ShowEnablePort=on  SampleTime=1
      settings: InputPortMap=u0,e6
  cfblk5 : simulink/Discrete/Transfer Fcn First Order  PoleZ=0.95  ICPrevOutput=0.0  DoSatur=off
  cfblk6 : Reshape
  cfblk7 : ComplexToRealImag
  cfblk8 : Trigonometry
  cfblk9 : Polyval  Coefs=[ +2.081618890e-019, -1.441693666e-014, +4.719686976e-010, -8.536869453e-006, +1.621573104e-001, -8.087801117e+001 ]
  cyemi_{450..459} (10 alike) : DataTypeConversion  OutDataTypeStr=double
  cfblk2 : Outport
  cfblk15 : Outport  Port=2
  cfblk16 : Outport  Port=3
  wires:
  cfblk8/1 -> cfblk2/1
  cfblk4/1 -> cfblk16/1
  cfblk11/1 -> cfblk15/1
  cyemi_450/1 -> cfblk10/1
  cfblk13/1 -> cyemi_450/1
  cyemi_451/1 -> cfblk17/1
  cfblk9/1 -> cyemi_451/1
  cyemi_452/1 -> cfblk3/1
  cfblk17/1 -> cyemi_452/1
  cyemi_453/1 -> cfblk4/1
  cfblk14/1 -> cyemi_453/1
  cyemi_454/1 -> cfblk4/2
  cfblk12/1 -> cyemi_454/1
  cyemi_455/1 -> cfblk5/1
  cfblk10/1 -> cyemi_455/1
  cyemi_456/1 -> cfblk6/1
  cfblk7/2 -> cyemi_456/1
  cyemi_457/1 -> cfblk7/1
  cfblk5/1 -> cyemi_457/1
  cyemi_458/1 -> cfblk8/1
  cfblk7/1 -> cyemi_458/1
  cyemi_459/1 -> cfblk9/1
  cfblk3/1 -> cyemi_459/1

== system sampleModel2120_pp_532_1/cfblk56/cfblk9 ==
  cfblk1 : Inport
  cfblk8 : Inport  Port=2
  cfblk9 : Inport  Port=3
  cfblk10 : Delay  SampleTime=1
  cfblk3 : Delay  DelayLengthSource=Input port  SampleTime=1
      settings: InputPortMap=u0,p1
  cfblk4 : Delay  SampleTime=1
  cfblk5 : UnitDelay  HasFrameUpgradeWarning=on
  cfblk6 : Squeeze
  cfblk7 : Gain  Gain=[79600041.215616]  OutDataTypeStr=double
  cyemi_{471..476} (6 alike) : DataTypeConversion  OutDataTypeStr=double
  cfblk2 : Outport
  wires:
  cfblk8/1 -> cfblk2/1
  cfblk4/1 -> cfblk6/1
  cyemi_471/1 -> cfblk10/1
  cfblk6/1 -> cyemi_471/1
  cyemi_472/1 -> cfblk3/1
  cfblk7/1 -> cyemi_472/1
  cyemi_473/1 -> cfblk3/2
  cfblk9/1 -> cyemi_473/1
  cyemi_474/1 -> cfblk4/1
  cfblk10/1 -> cyemi_474/1
  cyemi_475/1 -> cfblk5/1
  cfblk3/1 -> cyemi_475/1
  cyemi_476/1 -> cfblk7/1
  cfblk1/1 -> cyemi_476/1

== system sampleModel2120_pp_532_1/cfblk57/cfblk10 ==
  cfblk1 : Inport
  cfblk6 : Inport  Port=2
  cfblk7 : Inport  Port=3
  cfblk8 : Inport  Port=4
  cfblk3 : UnitDelay  HasFrameUpgradeWarning=on
  cfblk4 : Gain  Gain=[111519645.916665]  OutDataTypeStr=double
  cfblk5 : Reshape
  cyemi_482 : DataTypeConversion  OutDataTypeStr=double
  cyemi_483 : DataTypeConversion  OutDataTypeStr=double
  cyemi_484 : DataTypeConversion  OutDataTypeStr=double
  cfblk2 : Outport
  wires:
  cfblk4/1 -> cfblk2/1
  cyemi_482/1 -> cfblk3/1
  cfblk5/1 -> cyemi_482/1
  cyemi_483/1 -> cfblk4/1
  cfblk6/1 -> cyemi_483/1
  cyemi_484/1 -> cfblk5/1
  cfblk8/1 -> cyemi_484/1

== system sampleModel2120_pp_532_1/cfblk57/cfblk11 ==
  cfblk1 : Inport
  cfblk9 : Inport  Port=2
  cfblk10 : Delay  SampleTime=1
  cfblk3 : Delay  SampleTime=1
  cfblk4 : DiscreteStateSpace
  cfblk5 : simulink/Discrete/Transfer Fcn Lead or Lag  PoleZ=0.95  ZeroZ=0.75  ICPrevOutput=0.0  ICPrevInput=0.0  DoSatur=off
      settings: SourceProductBaseCode=SL
  cfblk6 : DiscreteZeroPole  Poles=[0 0.5]  Gain=1
  cfblk7 : Trigonometry
  cfblk8 : ComplexToRealImag
  cyemi_{487..493} (7 alike) : DataTypeConversion  OutDataTypeStr=double
  cfblk2 : Outport
  wires:
  cfblk8/2 -> cfblk2/1
  cyemi_487/1 -> cfblk10/1
  cfblk6/1 -> cyemi_487/1
  cyemi_488/1 -> cfblk3/1
  cfblk10/1 -> cyemi_488/1
  cyemi_489/1 -> cfblk4/1
  cfblk5/1 -> cyemi_489/1
  cyemi_490/1 -> cfblk5/1
  cfblk8/1 -> cyemi_490/1
  cyemi_491/1 -> cfblk6/1
  cfblk7/1 -> cyemi_491/1
  cyemi_492/1 -> cfblk7/1
  cfblk4/1 -> cyemi_492/1
  cyemi_493/1 -> cfblk8/1
  cfblk3/1 -> cyemi_493/1

== system sampleModel2120_pp_532_1/cfblk57/cfblk12 ==
  cfblk1 : Inport
  cfblk8 : Inport  Port=2
  cfblk3 : simulink/Discrete/Tapped Delay  vinit=0.0  samptime=-1  NumDelays=1  DelayOrder=Oldest  includeCurrent=off
  cfblk4 : Delay  DelayLengthSource=Input port  SampleTime=1
      settings: InputPortMap=u0,p1
  cfblk5 : Rounding
  cfblk6 : Sin  TimeSource=Use external signal  SampleTime=0
  cfblk7 : Bias  Bias=[-951001195.400587]
  cyemi_{496..501} (6 alike) : DataTypeConversion  OutDataTypeStr=double
  cfblk2 : Outport
  cfblk9 : Outport  Port=2
  wires:
  cfblk7/1 -> cfblk2/1
  cfblk5/1 -> cyemi_496/1, cyemi_498/1
  cfblk4/1 -> cfblk9/1
  cyemi_496/1 -> cfblk3/1
  cyemi_497/1 -> cfblk4/1
  cfblk6/1 -> cyemi_497/1
  cyemi_498/1 -> cfblk4/2
  cyemi_499/1 -> cfblk5/1
  cfblk1/1 -> cyemi_499/1
  cyemi_500/1 -> cfblk6/1
  cfblk3/1 -> cyemi_500/1
  cyemi_501/1 -> cfblk7/1
  cfblk8/1 -> cyemi_501/1

== system sampleModel2120_pp_532_1/cfblk57/cfblk13 ==
  cfblk1 : Inport
  cfblk7 : Inport  Port=2
  cfblk3 : simulink/Discrete/Transfer Fcn Real Zero  ZeroZ=0.75  ICPrevInput=0.0  DoSatur=off
      settings: SourceProductBaseCode=SL
  cfblk4 : Sum  Inputs=+-  OutDataTypeStr=double
  cfblk5 : Signum
  cfblk6 : Squeeze
  cyemi_{504..507} (4 alike) : DataTypeConversion  OutDataTypeStr=double
  cfblk2 : Outport
  wires:
  cfblk3/1 -> cfblk6/1
  cfblk6/1 -> cfblk2/1, cyemi_507/1
  cyemi_504/1 -> cfblk3/1
  cfblk4/1 -> cyemi_504/1
  cyemi_505/1 -> cfblk4/1
  cfblk1/1 -> cyemi_505/1
  cyemi_506/1 -> cfblk4/2
  cfblk7/1 -> cyemi_506/1
  cyemi_507/1 -> cfblk5/1

== system sampleModel2120_pp_532_1/cfblk57/cfblk14 ==
  cfblk1 : Inport
  cfblk6 : Inport  Port=2
  cfblk3 : Gain  Gain=[374890354.692374]  OutDataTypeStr=double
  cfblk4 : Sqrt  Operator=rSqrt  OutDataTypeStr=double  AlgorithmType=Newton-Raphson  SaturateOnIntegerOverflow=on
  cfblk5 : Product  Inputs=*  OutDataTypeStr=double
  cyemi_510 : DataTypeConversion  OutDataTypeStr=double
  cyemi_511 : DataTypeConversion  OutDataTypeStr=double
  cyemi_512 : DataTypeConversion  OutDataTypeStr=double
  cfblk2 : Outport
  cfblk7 : Outport  Port=2
  cfblk8 : Outport  Port=3
  wires:
  cfblk3/1 -> cfblk7/1
  cfblk1/1 -> cfblk8/1, cyemi_512/1
  cfblk4/1 -> cfblk2/1
  cyemi_510/1 -> cfblk3/1
  cfblk6/1 -> cyemi_510/1
  cyemi_511/1 -> cfblk4/1
  cfblk5/1 -> cyemi_511/1
  cyemi_512/1 -> cfblk5/1
